simulink model "LabFabSim2022a__10_6_2023"  (R2022a)
settings: Solver=VariableStepAuto  StartTime=0.0  StopTime=400  RelTol=1e-3  EnableMultiTasking=on
model workspace (MAT data in the model file):
  JsonData = timetable
  JsonData.any.CustomProps = struct()
  JsonData.any.VariableCustomProps = struct()
  JsonData.any.versionSavedFrom = 5
  JsonData.any.minCompatibleVersion = 2
  JsonData.any.incompatibilityMsg = ''
  JsonData.any.arrayProps.Description = ''
  JsonData.any.arrayProps.UserData = []
  JsonData.any.arrayProps.TableCustomProperties = struct()
  JsonData.any.data = {[1; 2; 3; 4; 5; 6; 7; 8; 9]}
  JsonData.any.numDims = 2
  JsonData.any.useVarNamesOrig = 0
  JsonData.any.useDimNamesOrig = 0
  JsonData.any.dimNames = {'Time', 'Variables'}
  JsonData.any.dimNamesOrig = {}
  JsonData.any.varNames = {'PartID'}
  JsonData.any.varNamesOrig = {}
  JsonData.any.numRows = 9
  JsonData.any.numVars = 1
  JsonData.any.varDescriptions = {}
  JsonData.any.varUnits = {}
  JsonData.any.rowTimes = datetime
  JsonData.any.rowTimes.data = [1661950057191; 1661949738947; 1661949738947; 1661949738947; 1661949738947; 1661949738947; 1661949738948; 1661949738948; 1661949738948]
  JsonData.any.varContinuity = {}
  M = Simulink.Parameter
  M.DataType = 'auto'
  M.Complexity = 'real'
  M.Dimensions = [0 0]
  ROS_trigger = 0
  SL_ROS_VariableLengthArrays_MaxSizes.CommonInfo.ArrayTruncateAction = 'EmitWarning'
  SL_ROS_VariableLengthArrays_MaxSizes.MsgTypeMap = containers.Map
  SL_ROS_VariableLengthArrays_MaxSizes.MsgTypeMap.serialization.keys = {'std_msgs/UInt32MultiArray', 'std_msgs/UInt64MultiArray', 'std_msgs/UInt8MultiArray'}
  SL_ROS_VariableLengthArrays_MaxSizes.MsgTypeMap.serialization.values{1}.PropertyName = 'Data'
  SL_ROS_VariableLengthArrays_MaxSizes.MsgTypeMap.serialization.values{1}.DataType = 'uint32'
  SL_ROS_VariableLengthArrays_MaxSizes.MsgTypeMap.serialization.values{1}.MaxLength = 31
  SL_ROS_VariableLengthArrays_MaxSizes.MsgTypeMap.serialization.values{2}.PropertyName = 'Data'
  SL_ROS_VariableLengthArrays_MaxSizes.MsgTypeMap.serialization.values{2}.DataType = 'double'
  SL_ROS_VariableLengthArrays_MaxSizes.MsgTypeMap.serialization.values{2}.MaxLength = 31
  SL_ROS_VariableLengthArrays_MaxSizes.MsgTypeMap.serialization.values{3}.PropertyName = 'Data'
  SL_ROS_VariableLengthArrays_MaxSizes.MsgTypeMap.serialization.values{3}.DataType = 'uint8'
  SL_ROS_VariableLengthArrays_MaxSizes.MsgTypeMap.serialization.values{3}.MaxLength = 5
  SL_ROS_VariableLengthArrays_MaxSizes.MsgTypeMap.serialization.uniformity = 0
  SL_ROS_VariableLengthArrays_MaxSizes.MsgTypeMap.serialization.keyType = 'char'
  SL_ROS_VariableLengthArrays_MaxSizes.MsgTypeMap.serialization.valueType = 'any'
undefined symbols (not defined in the file): DOS, DOSinitGen, DTP, DTPGen, DTPInitGen, EmptyLocFound, InitCobot, InitCobotReturn, InitializeSLD, InitLEGO, InitVGRproc2, m, MC, MCGen, MCInitGen, MO, MOGen, MOInitGen, n, NetScan, NetScanInitGen, OrderGen, Spying, SpyingInitGen, WS, WSGen, WSInitGen
libraries: sldelib x1
(part 1 of 4)
settings Model: SimulationMode=external  ExtModeEnableFloating=off  Creator=ise  LastModifiedBy=zdewardener
settings SolverCC: AutoInsertRateTranBlk=on
settings DataIOCC: ExternalInput=[JsonData]  SaveOutput=off
settings OptimizationCC: DefaultParameterBehavior=Inlined  InlineInvariantSignals=on  EnhancedBackFolding=on  PassReuseOutputArgsAs=Individual arguments  StateBitsets=on  DataBitsets=on  ZeroExternalMemoryAtStartup=off  ZeroInternalMemoryAtStartup=off  NoFixptDivByZeroProtection=on  LifeSpan=1  MaxStackSize=64  OptimizeBlockOrder=speed  DifferentSizesBufferReuse=on  EfficientTunableParamExpr=on
settings DebuggingCC: ParameterTunabilityLossMsg=error  UnconnectedInputMsg=warning  UnconnectedOutputMsg=warning  UnconnectedLineMsg=warning
settings HardwareCC: ProdBitPerPointer=32  ProdBitPerSizeT=32  ProdBitPerPtrDiffT=32  ProdLargestAtomicFloat=None  ProdIntDivRoundTo=Floor  ProdWordSize=32  ProdHWDeviceType=Generic->Custom
settings RTWCC: SystemTargetFile=ert.tlc  HardwareBoard=Robot Operating System (ROS)  TLCOptions=-p0 -aRateBasedStepFcn=0  TemplateMakefile=ert_default_tmf  GenerateReport=on  RTWVerbose=off  Toolchain=Catkin  IncludeHyperlinkInReport=on  LaunchReport=on  DLArmComputeVersion=19.05
settings CodeAppCC: ForceParamTrailComments=on  IgnoreCustomStorageClasses=off  OperatorAnnotations=on  SimulinkDataObjDesc=on  SFDataObjDesc=on  CustomSymbolStrGlobalVar=rt$N$M  CustomSymbolStrType=$N$M  CustomSymbolStrFcn=$N$M$F  CustomSymbolStrMacro=$N$M  InsertBlockDesc=on
settings ERTTargetCC: TargetLangStandard=C99 (ISO)  CodeReplacementLibrary=ISO_C  SuppressErrorStatus=on  SupportAbsoluteTime=off  PurelyIntegerCode=on  SupportNonFinite=off  SupportComplex=off  InlinedParameterPlacement=NonHierarchical  RootIOFormat=Structure reference  ERTCustomFileTemplate=example_file_process.tlc

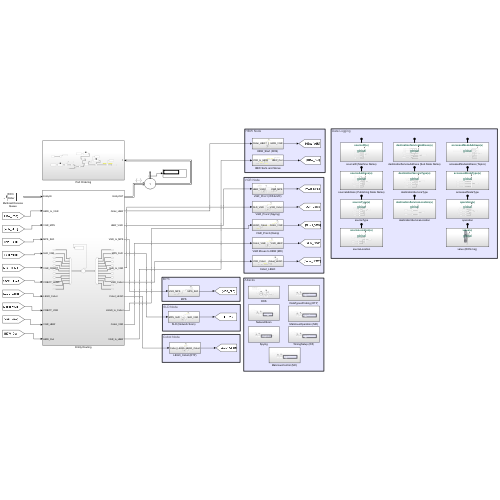
[thumbnail: Simulink's stored preview of the top-level diagram]
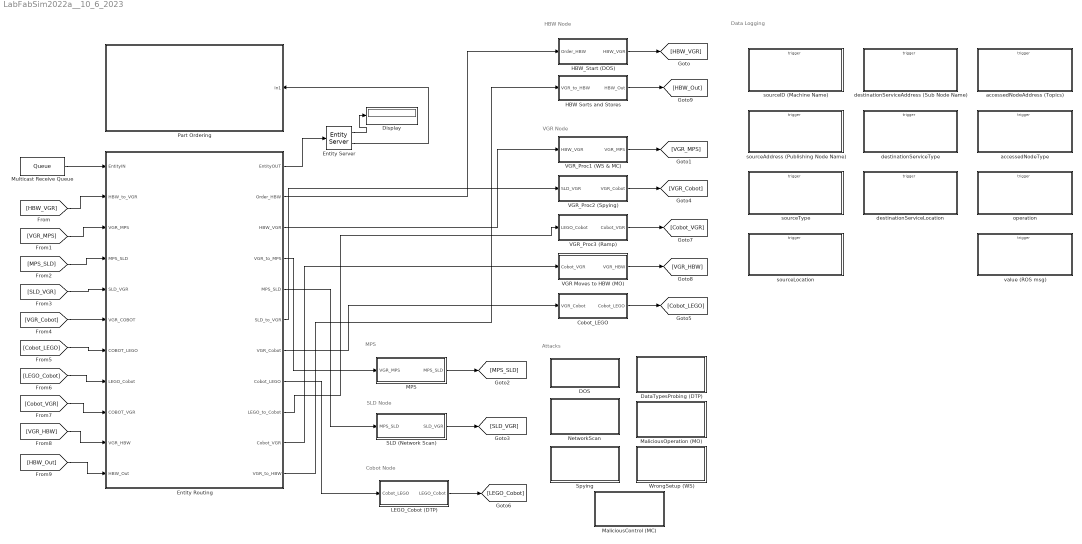
== system LabFabSim2022a__10_6_2023 ==
  note: Attacks
  note: Data Logging
  note: MPS
  note: Cobot Node
  note: SLD Node
  note: VGR Node
  note: HBW Node
  Cobot_LEGO : Subsystem
  DOS : Subsystem
  DataTypesProbing (DTP) : Subsystem
  Display : Display
  Entity Routing : Subsystem
  Entity Server : EntityServer  InputPortMessageModes=m  OutputPortMessageModes=n,m  Capacity=1  EntryAction=|  NumberEntitiesDeparted=on
      | %EntityGen();
      | ReleaseEntity();
      | 
      | entity.CurrentStep = 1;
      | entity.CurrentRoute = 1;
      settings: OutputPortMap=o0,o9
  HBW Sorts and Stores : Subsystem
  HBW_Start (DOS) : Subsystem
  LEGO_Cobot (DTP) : Subsystem
  MPS : Subsystem
  MaliciousControl (MC) : Subsystem
  MaliciousOperation (MO) : Subsystem
  Multicast Receive Queue : Queue  OutputPortMessageModes=m  Capacity=1  EntityArrivalSource=Multicast  MulticastTag=Order
  NetworkScan : Subsystem
  Part Ordering : Subsystem
      settings: PortSchema="{\"entries\":[{\"content\":{\"sides\":[{\"content\":{\"connectorIds\":[]},\"type\":\"ConnectorPlacement.EquallySpacedRectSide\",\"uuid\":\"e994c97d-fb45-4def-b0cb-77e379a9fe28\"},{\"content\":{\"connectorIds\":[\"In1\"],\"side\":\"RIGHT\"},\"type\":\"ConnectorPlacement.EquallySpacedRectSide\",\"uuid\":\"06ce1dc3-22b9-49bf-9481-b353835a56bd\"},{\"content\":{\"connectorIds\":[],\"side\":\"TOP\"},\"type\":\"ConnectorPlacement.EquallySpacedRectSide\",\"uuid\":\"0c5932e5-656f-479c-b83f-b876107c2f45\"}]},\"type\":\"ConnectorPlacement.EquallySpacedConnector\",\"uuid\":\"592d17c9-c3fc-48ea-a782-1c7751a95675\"}],\"packageUris\":[\"http://schema.mathworks.com/mf0/Connector/R2020b\"],\"version\":\"1.0\"}"
  SLD (Network Scan) : Subsystem
  Spying : Subsystem
  VGR Moves to HBW (MO) : Subsystem
  VGR_Proc1 (WS & MC) : Subsystem
  VGR_Proc2 (Spying) : Subsystem
  VGR_Proc3 (Ramp) : Subsystem
  WrongSetup (WS) : Subsystem
  accessedNodeAddress (Topics) : Subsystem  TreatAsAtomicUnit=on
  accessedNodeType : Subsystem  TreatAsAtomicUnit=on
  destinationServiceAddress (Sub Node Name) : Subsystem  TreatAsAtomicUnit=on
  destinationServiceLocation : Subsystem  TreatAsAtomicUnit=on
  destinationServiceType : Subsystem  TreatAsAtomicUnit=on
  operation : Subsystem  TreatAsAtomicUnit=on
  sourceAddress (Publishing Node Name) : Subsystem  TreatAsAtomicUnit=on
  sourceID (Machine Name) : Subsystem  TreatAsAtomicUnit=on
  sourceLocation : Subsystem  TreatAsAtomicUnit=on
  sourceType : Subsystem  TreatAsAtomicUnit=on
  value (ROS msg) : Subsystem  TreatAsAtomicUnit=on
  wires:
  Entity Server/1 -> Display/1
  [HBW_VGR] -> Entity Routing/2(HBW_to_VGR)
  [VGR_MPS] -> Entity Routing/3(VGR_MPS)
  [MPS_SLD] -> Entity Routing/4(MPS_SLD)
  [SLD_VGR] -> Entity Routing/5(SLD_VGR)
  [VGR_Cobot] -> Entity Routing/6(VGR_COBOT)
  [Cobot_LEGO] -> Entity Routing/7(COBOT_LEGO)
  Entity Routing/2(Order_HBW) -> HBW_Start (DOS)/1(Order_HBW)
  Entity Routing/4(VGR_to_MPS) -> MPS/1(VGR_MPS)
  Entity Routing/5("MPS_SLD ") -> SLD (Network Scan)/1(MPS_SLD)
  Entity Routing/6(SLD_to_VGR) -> VGR_Proc2 (Spying)/1(SLD_VGR)
  Entity Routing/7(VGR_Cobot) -> Cobot_LEGO/1(VGR_Cobot)
  HBW_Start (DOS)/1(HBW_VGR) -> [HBW_VGR]
  MPS/1(MPS_SLD) -> [MPS_SLD]
  SLD (Network Scan)/1(SLD_VGR) -> [SLD_VGR]
  VGR_Proc2 (Spying)/1(VGR_Cobot) -> [VGR_Cobot]
  Cobot_LEGO/1(Cobot_LEGO) -> [Cobot_LEGO]
  Entity Routing/3("HBW_VGR ") -> VGR_Proc1 (WS & MC)/1(HBW_VGR)
  VGR_Proc1 (WS & MC)/1(VGR_MPS) -> [VGR_MPS]
  Entity Routing/8(Cobot_LEGO) -> LEGO_Cobot (DTP)/1(Cobot_LEGO)
  [LEGO_Cobot] -> Entity Routing/8(LEGO_Cobot)
  LEGO_Cobot (DTP)/1(LEGO_Cobot) -> [LEGO_Cobot]
  Entity Routing/9(LEGO_to_Cobot) -> VGR_Proc3 (Ramp)/1(LEGO_Cobot)
  VGR_Proc3 (Ramp)/1(Cobot_VGR) -> [Cobot_VGR]
  [Cobot_VGR] -> Entity Routing/9(COBOT_VGR)
  Entity Routing/10(Cobot_VGR) -> VGR Moves to HBW (MO)/1(Cobot_VGR)
  [VGR_HBW] -> Entity Routing/10(VGR_HBW)
  VGR Moves to HBW (MO)/1(VGR_HBW) -> [VGR_HBW]
  Entity Routing/11(VGR_to_HBW) -> HBW Sorts and Stores/1(VGR_to_HBW)
  [HBW_Out] -> Entity Routing/11(HBW_Out)
  HBW Sorts and Stores/1(HBW_Out) -> [HBW_Out]
  Entity Server/2 -> Part Ordering/1(In1)
  Entity Routing/1(EntityOUT) -> Entity Server/1
  Multicast Receive Queue/1 -> Entity Routing/1(EntityIN)

== system LabFabSim2022a__10_6_2023/Cobot_LEGO ==
  note: Calling cobot for picking
  note: Order is ready for pickup
  VGR_Cobot : Inport
  Cobot moving to pickup loc : EntityServer  InputPortMessageModes=m  OutputPortMessageModes=m  Capacity=1  ServiceTimeSource=MATLAB action  ServiceTimeValue=0.1  ServiceTimeAction=|  EntryAction=|  ExitAction=|
      ServiceTimeAction=|
      | dt=0
      | persistent rngInit;
      | if isempty(rngInit)
      |     seed = entity.Rand_seed;
      |     rng(seed);
      |     rngInit = true;
      | end
      | 
      | if entity.ColorID == 1 %red
      |     % Pattern: Uniform distribution
      |     % m: Minimum, M: Maximum
      |     m = 0.2372; M = 0.2624;
      |     dt = m + (M - m) * rand;
      | elseif entity.ColorID == 2 %blue
      |     m = 0.1684; M = 0.2499;
      |     dt = m + (M - m) * rand;
      | elseif entity.ColorID == 3 %white
      |     m = 0.2056; M = 0.2679;
      |     dt = m + (M - m) * rand;
      | end
      EntryAction=|
      | sourceID(6); %cobot
      | sourceAddress(5); %/listener(cobot)
      | sourceType(1); %motion sensor
      | sourceLocation(1); %Fischertechnik
      | destinationServiceAddress(3); %/status_update(main)?
      | destinationServiceType(5); %Next task
      | destinationServiceLocation(2); %Expansion
      | accessedNodeAddress(5); 
      | accessedNodeType(2); %Boolean
      | operation(3); %notify-callback
      | value(34); %Order is ready for pickup
      ExitAction=|
      | sourceID(2); %vgr
      | sourceAddress(2); %/vgr_node
      | sourceType(1); %motion sensor
      | sourceLocation(1); %Fischertechnik
      | destinationServiceAddress(5); %/listener(cobot)
      | destinationServiceType(5); %next task
      | destinationServiceLocation(2); %Expansion
      | accessedNodeAddress(3); 
      | accessedNodeType(1); %String
      | operation(3); %notify-callback
      | value(33); %Calling cobot for picking
  Entity Gate : EntityGate  InputPortMessageModes=m,m  OutputPortMessageModes=m  OperatingMode=Release gate
  Entity Server : EntityServer  InputPortMessageModes=m  OutputPortMessageModes=m  Capacity=1  ServiceTimeSource=MATLAB action  ServiceTimeAction=|
      | dt=0
      | persistent rngInit;
      | if isempty(rngInit)
      |     seed = entity.Rand_seed;
      |     rng(seed);
      |     rngInit = true;
      | end
      | 
      | if entity.ColorID == 1 %red
      |     % Pattern: Uniform distribution
      |     % m: Minimum, M: Maximum
      |     m = 0.0028; M = 0.01;
      |     dt = m + (M - m) * rand;
      | elseif entity.ColorID == 2 %blue
      |     m = 0.007; M = 0.051;
      |     dt = m + (M - m) * rand;
      | elseif entity.ColorID == 3 %white
      |     m = 0.0037; M = 0.0045;
      |     dt = m + (M - m) * rand;
      | end
  Pump off; Return to home pos : EntityServer  InputPortMessageModes=m  OutputPortMessageModes=m  Capacity=1  ServiceTimeValue=5  EntryAction=InitLEGO();
  Pump on; Moving to main LEGO belt : EntityServer  InputPortMessageModes=m  OutputPortMessageModes=m  Capacity=1  ServiceTimeValue=15
  Simulink Function : Subsystem  TreatAsAtomicUnit=on
  Cobot_LEGO : Outport
  wires:
  VGR_Cobot/1 -> Entity Server/1
  Cobot moving to pickup loc/1 -> Pump on; Moving to main LEGO belt/1
  Pump on; Moving to main LEGO belt/1 -> Pump off; Return to home pos/1
  Pump off; Return to home pos/1 -> Entity Gate/2
  Entity Gate/1 -> Cobot_LEGO/1
  Simulink Function/1(Out1) -> Entity Gate/1
  Entity Server/1 -> Cobot moving to pickup loc/1

== system LabFabSim2022a__10_6_2023/DOS ==
  note: Entity Gate:
      | set to open when a positive signal value is passed into the control port. Closes when negative.
  note: Generates a single entity that causes DOSattack (entity generator) to generate 400 entities for DOS attack
  note: Sets DOS_id up to 400 and resets to 1 for next DOS attack
  note: On Service Completion: Send a signal to data-logging SimFunctions
  note: Service Time: 1 Timestep
  note: Recieve signal from Chance-setting Server block for activation signal
  DOS : Subsystem  TreatAsAtomicUnit=on
  Display : Display
  Entity Gate : EntityGate  InputPortMessageModes=m,m  OutputPortMessageModes=m
  Entity Generator : EntityGenerator  InputPortMessageModes=m  OutputPortMessageModes=m  GenerationMethod=Event-based  IntergenerationTimeAction=|  GenerateAction=|  AttributeName=DOS_id  EntityType=Structured  EntityTypeName=DOSattack
      IntergenerationTimeAction=|
      | chanceDOS = rand(1,1);
      | if chanceDOS < 0.3
      |     dt = 1
      GenerateAction=|
      | persistent next_id_DOS
      | 
      | if isempty(next_id_DOS)
      |     next_id_DOS = 1;
      |     %set seed for random number generation
      |     rng(12345);
      | end
      | 
      | entity.DOS_id = next_id_DOS
      | next_id_DOS = next_id_DOS + 1
      | 
      | if entity.DOS_id == 400
      |     next_id_DOS = 1
      settings: InputPortMap=u0
  Entity Server : EntityServer  InputPortMessageModes=m  OutputPortMessageModes=m  Capacity=1  ServiceTimeValue=1  ServiceCompleteAction=|
      | sourceID(3); %main
      | sourceAddress(6); %/order
      | sourceType(4); %order
      | sourceLocation(3); %SCADA system
      | destinationServiceAddress(1); %/hbw_node
      | destinationServiceType(4); %order
      | destinationServiceLocation(1); %Fischertechnik
      | accessedNodeAddress(1); 
      | accessedNodeType(1); %String
      | operation(3); %notify-callback
      | value(1); %hbw recieved an order
  Entity Store : EntityStore  InputPortMessageModes=m  OutputPortMessageModes=m  Capacity=401
      settings: OutputPortMap=o4
  Entity Terminator1 : EntityTerminator  InputPortMessageModes=m  NumberEntitiesArrived=on
      settings: OutputPortMap=o0
  InitDOS : Subsystem
  "Number of Entities Generated from main " : Display
  Simulink Function1 : Subsystem  TreatAsAtomicUnit=on
  Subsystem1 : Subsystem
  wires:
  InitDOS/1(Out1) -> "Number of Entities Generated from main "/1
  Subsystem1/1(Out1) -> Simulink Function1/1(In1)
  DOS/1(Out1) -> Entity Gate/1
  Entity Gate/1 -> Entity Server/1
  Entity Generator/1 -> Entity Store/1
  Entity Server/1 -> Entity Terminator1/1
  Simulink Function1/1(Out1) -> Entity Generator/1
  Entity Store/1 -> Entity Gate/2
  Entity Terminator1/1 -> Display/1

== system LabFabSim2022a__10_6_2023/DataTypesProbing (DTP) ==
  note: SourID(5), SourAdd(4), SourType(1), SourLoc(2), Dest.Serv.Add(5), Dest.Serv.Type(5), Dest.Serv.Loc(2), Acc.Node.Add(4), Acc.Node.Type(1,3), Op(1), Val(46)
  note: Entity Gate:
      | set to open when a positive signal value is passed into the control port. Closes when negative.
  note: Recieve signal from Chance-setting Server block for activation signal
  note: Service Time: 1000 Timestep
  note: Generates a single entity that causes Spying attack (entity generator) to generate one entity
  note: Sets DTP_id up to 6 and resets to 1 for next DataTypesProbing attack
  note: On Service Completion: Send a signal to data-logging SimFunctions
  note: Service Time: 310 Timestep
  Display : Display
  Entity Gate : EntityGate  InputPortMessageModes=m,m  OutputPortMessageModes=m
  Entity Generator : EntityGenerator  InputPortMessageModes=m  OutputPortMessageModes=m  GenerationMethod=Event-based  IntergenerationTimeAction=|  GenerateAction=|  AttributeName=DTP_id  EntityType=Structured  EntityTypeName=DTPAttack
      IntergenerationTimeAction=|
      | chanceDOS = rand(1,1);
      | if chanceDOS < 0.3
      |     dt = 1
      GenerateAction=|
      | persistent next_id_DTP
      | 
      | if isempty(next_id_DTP)
      |     next_id_DTP = 1;
      |     %set seed for random number generation
      |     rng(12345);
      | end
      | 
      | entity.DTP_id = next_id_DTP
      | next_id_DTP = next_id_DTP + 1
      | 
      | if entity.DTP_id == 1
      |     next_id_DTP = 1
      settings: InputPortMap=u0
  Entity Server : EntityServer  InputPortMessageModes=m  OutputPortMessageModes=m  Capacity=1  ServiceTimeValue=1000  ServiceCompleteAction=|
      | sourceID(5); %Lego
      | sourceAddress(1); %/lego_node
      | sourceType(1); %motion Sensor
      | sourceLocation(2); %Expansion
      | destinationServiceAddress(5); %/listener(cobot)
      | destinationServiceType(5); %Next Task
      | destinationServiceLocation(2); %Expansion
      | accessedNodeAddress(4); 
      | accessedNodeType(1); %String
      | operation(1); %read/write
      | value(46); %DTP
  Entity Server1 : EntityServer  InputPortMessageModes=m  OutputPortMessageModes=m  Capacity=1  ServiceTimeValue=310  ServiceCompleteAction=|
      | sourceID(5); %Lego
      | sourceAddress(1); %/lego_node
      | sourceType(1); %motion Sensor
      | sourceLocation(2); %Expansion
      | destinationServiceAddress(5); %/listener(cobot)
      | destinationServiceType(5); %Next Task
      | destinationServiceLocation(2); %Expansion
      | accessedNodeAddress(4); 
      | accessedNodeType(3); %Integer
      | operation(1); %read/write
      | value(46); %DTP
  Entity Store : EntityStore  InputPortMessageModes=m  OutputPortMessageModes=m  Capacity=2
      settings: OutputPortMap=o4
  Entity Terminator1 : EntityTerminator  InputPortMessageModes=m  NumberEntitiesArrived=on
      settings: OutputPortMap=o0
  InitDataTypesProbing : Subsystem
  "Number of Entities Generated from main " : Display
  Simulink Function1 : Subsystem  TreatAsAtomicUnit=on
  Spying : Subsystem  TreatAsAtomicUnit=on
  Subsystem1 : Subsystem
  wires:
  Simulink Function1/1(Out1) -> Entity Generator/1
  Entity Terminator1/1 -> Display/1
  Entity Generator/1 -> Entity Store/1
  Entity Store/1 -> Entity Gate/2
  Entity Server/1 -> Entity Server1/1
  Spying/1(Out1) -> Entity Gate/1
  Subsystem1/1(Out1) -> Simulink Function1/1(In1)
  InitDataTypesProbing/1(Out1) -> "Number of Entities Generated from main "/1
  Entity Server1/1 -> Entity Terminator1/1
  Entity Gate/1 -> Entity Server/1

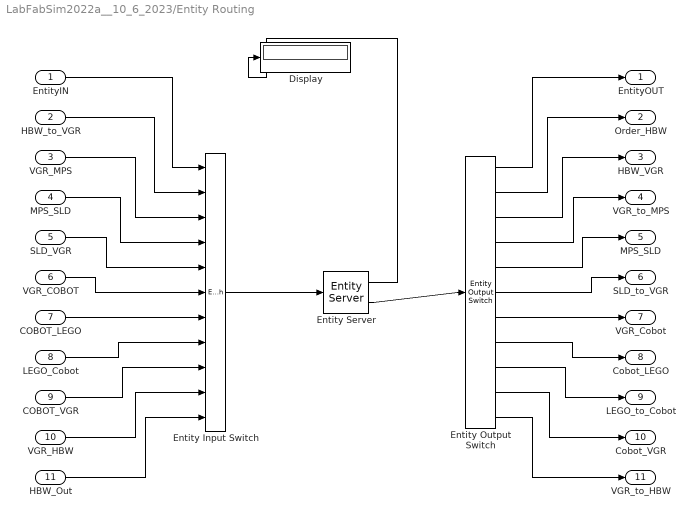
== system LabFabSim2022a__10_6_2023/Entity Routing ==
  EntityIN : Inport
  HBW_to_VGR : Inport  Port=2
  VGR_MPS : Inport  Port=3
  MPS_SLD : Inport  Port=4
  SLD_VGR : Inport  Port=5
  VGR_COBOT : Inport  Port=6
  COBOT_LEGO : Inport  Port=7
  LEGO_Cobot : Inport  Port=8
  COBOT_VGR : Inport  Port=9
  VGR_HBW : Inport  Port=10
  HBW_Out : Inport  Port=11
  Display : Display
  Entity Input Switch : EntityInputSwitch  InputPortMessageModes=m,m,m,m,m,m,m,m,m,m,m  OutputPortMessageModes=m  NumberInputPorts=11
      settings: InputPortMap=u1,u2,u3,u4,u5,u6,u7,u8,u9,u10,u11
  Entity Output Switch : EntityOutputSwitch  InputPortMessageModes=m  OutputPortMessageModes=m,m,m,m,m,m,m,m,m,m,m  NumberOutputPorts=11  SwitchingCriterion=From attribute  SwitchAttributeName=CurrentRoute
      settings: OutputPortMap=o0,o1,o2,o3,o4,o5,o6,o7,o8,o9,o10
  Entity Server : EntityServer  InputPortMessageModes=m  OutputPortMessageModes=n,m  Capacity=1  ServiceTimeValue=0  EntryAction=|  NumberEntitiesDeparted=on
      | entity.CurrentRoute = entity.ServiceProcess(entity.CurrentStep);
      | entity.CurrentStep = entity.CurrentStep + 1;
      settings: OutputPortMap=o0,o9
  EntityOUT : Outport
  Order_HBW : Outport  Port=2
  "HBW_VGR " : Outport  Port=3
  VGR_to_MPS : Outport  Port=4
  "MPS_SLD " : Outport  Port=5
  SLD_to_VGR : Outport  Port=6
  VGR_Cobot : Outport  Port=7
  Cobot_LEGO : Outport  Port=8
  LEGO_to_Cobot : Outport  Port=9
  Cobot_VGR : Outport  Port=10
  VGR_to_HBW : Outport  Port=11
  wires:
  EntityIN/1 -> Entity Input Switch/1
  HBW_to_VGR/1 -> Entity Input Switch/2
  VGR_MPS/1 -> Entity Input Switch/3
  MPS_SLD/1 -> Entity Input Switch/4
  SLD_VGR/1 -> Entity Input Switch/5
  VGR_COBOT/1 -> Entity Input Switch/6
  COBOT_LEGO/1 -> Entity Input Switch/7
  Entity Input Switch/1 -> Entity Server/1
  Entity Server/2 -> Entity Output Switch/1
  Entity Output Switch/1 -> EntityOUT/1
  Entity Output Switch/2 -> Order_HBW/1
  Entity Output Switch/3 -> "HBW_VGR "/1
  Entity Output Switch/4 -> VGR_to_MPS/1
  Entity Output Switch/5 -> "MPS_SLD "/1
  Entity Output Switch/6 -> SLD_to_VGR/1
  Entity Output Switch/7 -> VGR_Cobot/1
  Entity Server/1 -> Display/1
  Entity Output Switch/8 -> Cobot_LEGO/1
  Entity Output Switch/9 -> LEGO_to_Cobot/1
  Entity Output Switch/10 -> Cobot_VGR/1
  Entity Output Switch/11 -> VGR_to_HBW/1
  LEGO_Cobot/1 -> Entity Input Switch/8
  COBOT_VGR/1 -> Entity Input Switch/9
  VGR_HBW/1 -> Entity Input Switch/10
  HBW_Out/1 -> Entity Input Switch/11

== system LabFabSim2022a__10_6_2023/HBW Sorts and Stores ==
  note: HBW Robot is Set to Home
  note: Status updated successfully
  note: HBW Placed Material on the Shelf
  note: VGR is Set to Home
  note: HBW Picked up Material from the Belt
  note: Material is Ready for HBW Pick Up
  VGR_to_HBW : Inport
  Entity Server : EntityServer  InputPortMessageModes=m  OutputPortMessageModes=m  Capacity=1  ServiceTimeSource=MATLAB action  ServiceTimeAction=|
      | dt=0
      | persistent rngInit;
      | if isempty(rngInit)
      |     seed = entity.Rand_seed;
      |     rng(seed);
      |     rngInit = true;
      | end
      | 
      | if entity.ColorID == 1 %red
      |     % Pattern: Uniform distribution
      |     % m: Minimum, M: Maximum
      |     m = 1.9949; M = 1.9965;
      |     dt = m + (M - m) * rand;
      | elseif entity.ColorID == 2 %blue
      |     m = 1.9508; M = 1.9938;
      |     dt = m + (M - m) * rand;
      | elseif entity.ColorID == 3 %white
      |     m = 1.8972; M = 1.9967;
      |     dt = m + (M - m) * rand;
      | end
  Entity Server1 : EntityServer  InputPortMessageModes=m  OutputPortMessageModes=m  Capacity=1  ServiceTimeSource=MATLAB action  ServiceTimeAction=|
      | dt=0
      | persistent rngInit;
      | if isempty(rngInit)
      |     seed = entity.Rand_seed;
      |     rng(seed);
      |     rngInit = true;
      | end
      | 
      | if entity.ColorID == 1 %red
      |     % Pattern: Uniform distribution
      |     % m: Minimum, M: Maximum
      |     m = 19.7937; M = 19.8988;
      |     dt = m + (M - m) * rand;
      | elseif entity.ColorID == 2 %blue
      |     m = 16.4596; M = 16.7641;
      |     dt = m + (M - m) * rand;
      | elseif entity.ColorID == 3 %white
      |     m = 23.1035; M = 23.7903;
      |     dt = m + (M - m) * rand;
      | end
  HBW Sorting and updating json file : EntityServer  InputPortMessageModes=m  OutputPortMessageModes=m  Capacity=1  ServiceTimeSource=MATLAB action  ServiceTimeValue=0.5  ServiceTimeAttributeName=HBW_ServiceTime  ServiceTimeAction=|  EntryAction=|  ExitAction=|
      ServiceTimeAction=|
      | dt=0
      | persistent rngInit;
      | if isempty(rngInit)
      |     seed = entity.Rand_seed;
      |     rng(seed);
      |     rngInit = true;
      | end
      | 
      | if entity.ColorID == 1 %red
      |     % Pattern: Uniform distribution
      |     % m: Minimum, M: Maximum
      |     m = 0.0103; M = 0.0276;
      |     dt = m + (M - m) * rand;
      | elseif entity.ColorID == 2 %blue
      |     m = 0.0071; M = 0.0138;
      |     dt = m + (M - m) * rand;
      | elseif entity.ColorID == 3 %white
      |     m = 0.014; M = 0.0204;
      |     dt = m + (M - m) * rand;
      | end
      EntryAction=|
      | sourceID(1); %hbw
      | sourceAddress(1); %/hbw_node
      | sourceType(5); %next task
      | sourceLocation(1); %Fischertechnik
      | destinationServiceAddress(3); %/status_update
      | destinationServiceType(5); %next task
      | destinationServiceLocation(1); %Fischertechnik
      | accessedNodeAddress(1); 
      | accessedNodeType(1); %String
      | operation(3); %notify-callback
      | value(14); %hbw empty box is back on the shelf
      ExitAction=|
      | sourceID(1); %hbw
      | sourceAddress(1); %/hbw_node
      | sourceType(5); %next task
      | sourceLocation(1); %Fischertechnik
      | destinationServiceAddress(3); %/status_update
      | destinationServiceType(5); %next task
      | destinationServiceLocation(1); %Fischertechnik
      | accessedNodeAddress(6); 
      | accessedNodeType(1); %String
      | operation(3); %notify-callback
      | value(42); %Status Updated Successfully
  HBW returns home : EntityServer  InputPortMessageModes=m  OutputPortMessageModes=m  Capacity=1  ServiceTimeSource=MATLAB action  ServiceTimeValue=20  ServiceTimeAttributeName=HBW_ServiceTime  ServiceTimeAction=|  ExitAction=|
      ServiceTimeAction=|
      | dt=0
      | persistent rngInit;
      | if isempty(rngInit)
      |     seed = entity.Rand_seed;
      |     rng(seed);
      |     rngInit = true;
      | end
      | 
      | if entity.ColorID == 1 %red
      |     % Pattern: Uniform distribution
      |     % m: Minimum, M: Maximum
      |     m = 14.049; M = 14.2335;
      |     dt = m + (M - m) * rand;
      | elseif entity.ColorID == 2 %blue
      |     m = 10.9437; M = 11.1714;
      |     dt = m + (M - m) * rand;
      | elseif entity.ColorID == 3 %white
      |     m = 17.375; M = 17.9006;
      |     dt = m + (M - m) * rand;
      | end
      ExitAction=|
      | sourceID(1); %hbw
      | sourceAddress(1); %/hbw_node
      | sourceType(3); %reference switch
      | sourceLocation(1); %Fischertechnik
      | destinationServiceAddress(3); %/status_update
      | destinationServiceType(5); %next task
      | destinationServiceLocation(1); %Fischertechnik
      | accessedNodeAddress(1); 
      | accessedNodeType(1); %String
      | operation(3); %notify-callback
      | value(15); %hbw robot is set to home
  "HBW-side light gate " : EntityServer  InputPortMessageModes=m  OutputPortMessageModes=m  Capacity=1  ServiceTimeSource=MATLAB action  ServiceTimeValue=0.5  ServiceTimeAttributeName=HBW_ServiceTime  ServiceTimeAction=|  EntryAction=|  ExitAction=|
      ServiceTimeAction=|
      | dt=0
      | persistent rngInit;
      | if isempty(rngInit)
      |     seed = entity.Rand_seed;
      |     rng(seed);
      |     rngInit = true;
      | end
      | 
      | if entity.ColorID == 1 %red
      |     % Pattern: Uniform distribution
      |     % m: Minimum, M: Maximum
      |     m = 0.5351; M = 0.5768;
      |     dt = m + (M - m) * rand;
      | elseif entity.ColorID == 2 %blue
      |     m = 0.5457; M = 0.5946;
      |     dt = m + (M - m) * rand;
      | elseif entity.ColorID == 3 %white
      |     m = 0.5429; M = 0.5509;
      |     dt = m + (M - m) * rand;
      | end
      EntryAction=|
      | sourceID(1); %hbw
      | sourceAddress(1); %/hbw_node
      | sourceType(1); %Motion Sensor
      | sourceLocation(1); %Fischertechnik
      | destinationServiceAddress(1); %/hbw_node
      | destinationServiceType(5); %next task
      | destinationServiceLocation(1); %Fischertechnik
      | accessedNodeAddress(1); 
      | accessedNodeType(2); %Boolean
      | operation(3); %notify-callback
      | value(10); %Material is Ready for HBW Pick Up
      ExitAction=|
      | sourceID(1); %hbw
      | sourceAddress(1); %/hbw_node
      | sourceType(1); %Motion Sensor
      | sourceLocation(1); %Fischertechnik
      | destinationServiceAddress(1); %/hbw_node
      | destinationServiceType(5); %next task
      | destinationServiceLocation(1); %Fischertechnik
      | accessedNodeAddress(1); 
      | accessedNodeType(2); %Boolean
      | operation(3); %notify-callback
      | value(12); %HBW Picked up Material from the Belt
  VGR returns home : EntityServer  InputPortMessageModes=m  OutputPortMessageModes=m  Capacity=1  ServiceTimeSource=MATLAB action  ServiceTimeValue=1.7  ServiceTimeAttributeName=HBW_ServiceTime  ServiceTimeAction=|  ServiceCompleteAction=|
      ServiceTimeAction=|
      | dt=0
      | persistent rngInit;
      | if isempty(rngInit)
      |     seed = entity.Rand_seed;
      |     rng(seed);
      |     rngInit = true;
      | end
      | 
      | if entity.ColorID == 1 %red
      |     % Pattern: Uniform distribution
      |     % m: Minimum, M: Maximum
      |     m = 1.4321; M = 1.478;
      |     dt = m + (M - m) * rand;
      | elseif entity.ColorID == 2 %blue
      |     m = 1.3652; M = 1.4388;
      |     dt = m + (M - m) * rand;
      | elseif entity.ColorID == 3 %white
      |     m = 1.3846; M = 1.45;
      |     dt = m + (M - m) * rand;
      | end
      ServiceCompleteAction=|
      | sourceID(2); %vgr
      | sourceAddress(2); %/vgr_node
      | sourceType(5); %next task
      | sourceLocation(1); %Fischertechnik
      | destinationServiceAddress(2); %/vgr_node
      | destinationServiceType(3); %reference switch
      | destinationServiceLocation(1); %Fischertechnik
      | accessedNodeAddress(3); 
      | accessedNodeType(1); %String
      | operation(3); %notify-callback
      | value(16); %vgr is set to home
  HBW_Out : Outport
  wires:
  VGR_to_HBW/1 -> Entity Server/1
  "HBW-side light gate "/1 -> VGR returns home/1
  Entity Server/1 -> "HBW-side light gate "/1
  VGR returns home/1 -> Entity Server1/1
  HBW Sorting and updating json file/1 -> HBW returns home/1
  HBW returns home/1 -> HBW_Out/1
  Entity Server1/1 -> HBW Sorting and updating json file/1

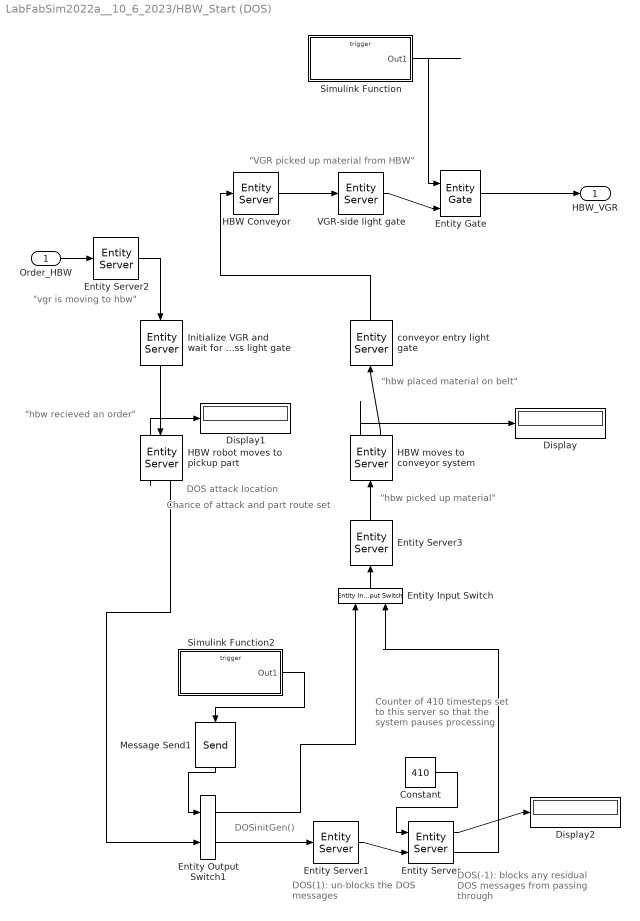
== system LabFabSim2022a__10_6_2023/HBW_Start (DOS) ==
  note: Chance of attack and part route set
  note: Counter of 410 timesteps set to this server so that the system pauses processing
  note: DOS(-1):
      | blocks any residual DOS messages from passing through
  note: DOS(1):
      | un-blocks the DOS messages
  note: "vgr is moving to hbw"
  note: "VGR picked up material from HBW"
  note: "hbw placed material on belt"
  note: "hbw picked up material"
  note: "hbw recieved an order"
  note: DOS attack location
  note: DOSinitGen()
  Order_HBW : Inport
  Constant : Constant  Value=410
  Display : Display
  Display1 : Display
  Display2 : Display
  Entity Input Switch : EntityInputSwitch  InputPortMessageModes=m,m  OutputPortMessageModes=m
  Entity Output Switch1 : EntityOutputSwitch  InputPortMessageModes=m,m  OutputPortMessageModes=m,m  SwitchingCriterion=From control port  SwitchAttributeName=Attribute1
      settings: InputPortMap=u0,u1
  Entity Gate : EntityGate  InputPortMessageModes=m,m  OutputPortMessageModes=m  OperatingMode=Release gate
  Entity Server : EntityServer  InputPortMessageModes=n,m  OutputPortMessageModes=n,m  Capacity=1  ServiceTimeSource=Signal port  ExitAction=DOS(-1);  NumberEntitiesDeparted=on
      settings: InputPortMap=u0,u2  OutputPortMap=o0,o9
  Entity Server1 : EntityServer  InputPortMessageModes=m  OutputPortMessageModes=m  Capacity=1  EntryAction=DOSinitGen();  ServiceCompleteAction=DOS(1);
  Entity Server2 : EntityServer  InputPortMessageModes=m  OutputPortMessageModes=m  Capacity=1  ServiceTimeSource=MATLAB action  ServiceTimeAction=|
      | dt=0
      | persistent rngInit;
      | if isempty(rngInit)
      |     seed = entity.Rand_seed;
      |     rng(seed);
      |     rngInit = true;
      | end
      | 
      | if entity.ColorID == 1 %red
      |     % Pattern: Uniform distribution
      |     % m: Minimum, M: Maximum
      |     m = 0.01819; M = 0.11747;
      |     dt = m + (M - m) * rand;
      | elseif entity.ColorID == 2 %blue
      |     m = 0.00819; M = 0.10134;
      |     dt = m + (M - m) * rand;
      | elseif entity.ColorID == 3 %white
      |     m = 0.00559; M = 0.05693;
      |     dt = m + (M - m) * rand;
      | end
  Entity Server3 : EntityServer  InputPortMessageModes=m  OutputPortMessageModes=m  Capacity=1  ServiceTimeSource=MATLAB action  ServiceTimeAction=|
      | dt=0
      | persistent rngInit;
      | if isempty(rngInit)
      |     seed = entity.Rand_seed;
      |     rng(seed);
      |     rngInit = true;
      | end
      | 
      | if entity.ColorID == 1 %red
      |     % Pattern: Uniform distribution
      |     % m: Minimum, M: Maximum
      |     m = 13.81674; M = 15.52105;
      |     dt = m + (M - m) * rand;
      | elseif entity.ColorID == 2 %blue
      |     m = 10.68302; M = 10.81544;
      |     dt = m + (M - m) * rand;
      | elseif entity.ColorID == 3 %white
      |     m = 17.46035; M = 18.19719;
      |     dt = m + (M - m) * rand;
      | end
  HBW Conveyor : EntityServer  InputPortMessageModes=m  OutputPortMessageModes=m  Capacity=1  ServiceTimeSource=MATLAB action  ServiceTimeAction=|
      | dt=0
      | persistent rngInit;
      | if isempty(rngInit)
      |     seed = entity.Rand_seed;
      |     rng(seed);
      |     rngInit = true;
      | end
      | 
      | if entity.ColorID == 1 %red
      |     % Pattern: Uniform distribution
      |     % m: Minimum, M: Maximum
      |     m = 4.91336; M = 4.93075;
      |     dt = m + (M - m) * rand;
      | elseif entity.ColorID == 2 %blue
      |     m = 5.01319; M = 5.07688;
      |     dt = m + (M - m) * rand;
      | elseif entity.ColorID == 3 %white
      |     m = 4.93141; M = 4.97213;
      |     dt = m + (M - m) * rand;
      | end
  HBW moves to conveyor system : EntityServer  InputPortMessageModes=m  OutputPortMessageModes=n,m  Capacity=1  ServiceTimeSource=MATLAB action  ServiceTimeValue=5  ServiceTimeAttributeName=HBW_ServiceTime  ServiceTimeAction=|  EntryAction=|  NumberEntitiesDeparted=on
      ServiceTimeAction=|
      | dt=0
      | persistent rngInit;
      | if isempty(rngInit)
      |     seed = entity.Rand_seed;
      |     rng(seed);
      |     rngInit = true;
      | end
      | 
      | if entity.ColorID == 1 %red
      |     % Pattern: Uniform distribution
      |     % m: Minimum, M: Maximum
      |     m = 18.6675; M = 20.17508;
      |     dt = m + (M - m) * rand;
      | elseif entity.ColorID == 2 %blue
      |     m = 17.17357; M = 17.69853;
      |     dt = m + (M - m) * rand;
      | elseif entity.ColorID == 3 %white
      |     m = 23.25977; M = 23.95334;
      |     dt = m + (M - m) * rand;
      | end
      EntryAction=|
      | sourceID(1); %hbw
      | sourceAddress(1); %/hbw_node
      | sourceType(3); %reference switch
      | sourceLocation(1); %Fischertechnik
      | destinationServiceAddress(1); %/hbw_node
      | destinationServiceType(5); %next task
      | destinationServiceLocation(1); %Fischertechnik
      | accessedNodeAddress(1); 
      | accessedNodeType(1); %String
      | operation(3); %notify-callback
      | value(3); %hbw picked up materials
      settings: OutputPortMap=o0,o9
  HBW robot moves to pickup part : EntityServer  InputPortMessageModes=m  OutputPortMessageModes=n,m  Capacity=1  ServiceTimeValue=0  ServiceTimeAttributeName=entity  EntryAction=|  ExitAction=|  NumberEntitiesDeparted=on
      EntryAction=|
      | sourceID(3); %main
      | sourceAddress(1); %/hbw_node
      | sourceType(4); %order
      | sourceLocation(3); %SCADA system
      | destinationServiceAddress(1); %/hbw_node
      | destinationServiceType(4); %order
      | destinationServiceLocation(1); %Fischertechnik
      | accessedNodeAddress(1); 
      | accessedNodeType(1); %String
      | operation(3); %notify-callback
      | value(1); %hbw recieved an order
      ExitAction=|
      | chanceDOS = rand(1,1)
      | if chanceDOS < 0.0
      |     %DOS Attack Happening!
      |     DOS_Router(1);
      | 
      | else
      |     %Normal Behavior
      |     DOS(-1);
      |     DOS_Router(2);
      | end
      settings: OutputPortMap=o0,o9
  Initialize VGR and wait for part to cross light gate : EntityServer  InputPortMessageModes=m  OutputPortMessageModes=m  Capacity=1  ServiceTimeSource=MATLAB action  ServiceTimeValue=0.2  ServiceTimeAction=|  EntryAction=|
      ServiceTimeAction=|
      | dt=0
      | persistent rngInit;
      | if isempty(rngInit)
      |     seed = entity.Rand_seed;
      |     rng(seed);
      |     rngInit = true;
      | end
      | 
      | if entity.ColorID == 1 %red
      |     % Pattern: Uniform distribution
      |     % m: Minimum, M: Maximum
      |     m = 0.00869; M = 0.01195;
      |     dt = m + (M - m) * rand;
      | elseif entity.ColorID == 2 %blue
      |     m = 0.00814; M = 0.11476;
      |     dt = m + (M - m) * rand;
      | elseif entity.ColorID == 3 %white
      |     m = 0.00951; M = 0.01176;
      |     dt = m + (M - m) * rand;
      | end
      EntryAction=|
      | sourceID(3); %main
      | sourceAddress(2); %/vgr_node
      | sourceType(5); %next task
      | sourceLocation(1); %Fischer
      | destinationServiceAddress(2); %/vgr_node
      | destinationServiceType(5); %next task
      | destinationServiceLocation(1); %Fischertechnik
      | accessedNodeAddress(3); 
      | accessedNodeType(1); %String
      | operation(3); %notify-callback
      | value(29); %vgr is moving to hbw
  Message Send1 : Send  OutputPortMessageModes=m
  Simulink Function : Subsystem  TreatAsAtomicUnit=on
  Simulink Function2 : Subsystem  TreatAsAtomicUnit=on
  VGR-side light gate : EntityServer  InputPortMessageModes=m  OutputPortMessageModes=m  Capacity=1  ServiceTimeValue=0.1  EntryAction=|
      | VGR_PickupPart();
      | 
      | sourceID(1); %hbw
      | sourceAddress(1); %/hbw_node
      | sourceType(1); %Motion Sensor 
      | sourceLocation(1); %Fischertechnik
      | destinationServiceAddress(2); %/vgr_node
      | destinationServiceType(5); %next task
      | destinationServiceLocation(1); %Fischertechnik
      | accessedNodeAddress(3); 
      | accessedNodeType(2); %Boolean
      | operation(3); %notify-callback
      | value(30); %VGR picked up material from HBW
  conveyor entry light gate : EntityServer  InputPortMessageModes=m  OutputPortMessageModes=m  Capacity=1  ServiceTimeValue=3  EntryAction=|
      | VGR_PickupPart();
      | 
      | sourceID(1); %hbw
      | sourceAddress(1); %/hbw_node
      | sourceType(1); %Motion Sensor
      | sourceLocation(1); %Fischertechnik
      | destinationServiceAddress(1); %/hbw_node
      | destinationServiceType(5); %next task
      | destinationServiceLocation(1); %Fischertechnik
      | accessedNodeAddress(1); 
      | accessedNodeType(1); %String
      | operation(3); %notify-callback
      | value(5); %hbw placed material on belt
  HBW_VGR : Outport
  wires:
  Simulink Function/1(Out1) -> Entity Gate/1
  Entity Gate/1 -> HBW_VGR/1
  HBW moves to conveyor system/2 -> conveyor entry light gate/1
  conveyor entry light gate/1 -> HBW Conveyor/1
  HBW Conveyor/1 -> VGR-side light gate/1
  VGR-side light gate/1 -> Entity Gate/2
  Order_HBW/1 -> Entity Server2/1
  Initialize VGR and wait for part to cross light gate/1 -> HBW robot moves to pickup part/1
  Entity Output Switch1/1 -> Entity Input Switch/1
  HBW moves to conveyor system/1 -> Display/1
  HBW robot moves to pickup part/1 -> Display1/1
  HBW robot moves to pickup part/2 -> Entity Output Switch1/2
  Entity Output Switch1/2 -> Entity Server1/1
  Entity Server/2 -> Entity Input Switch/2
  Entity Input Switch/1 -> Entity Server3/1
  Constant/1 -> Entity Server/1
  Simulink Function2/1(Out1) -> Message Send1/1
  Message Send1/1 -> Entity Output Switch1/1
  Entity Server/1 -> Display2/1
  Entity Server1/1 -> Entity Server/2
  Entity Server2/1 -> Initialize VGR and wait for part to cross light gate/1
  Entity Server3/1 -> HBW moves to conveyor system/1

== system LabFabSim2022a__10_6_2023/LEGO_Cobot (DTP) ==
  note: <color> order is ready for pickup
  note: DTP (1):
      | un-blocks the DataTypesProbing messages
  note: DTP(-1):
      | blocks any residual DataTypesProbing messages from passing through
  note: Counter of 11,311 timesteps set to this server so that the system pauses processing (1/10 of the time taken in DS2OS dataset)
  note: DTP InitGen()
  note: DataTypesProbing attack location
  note: Chance of attack and part route set
  Cobot_LEGO : Inport
  Constant : Constant  Value=1311
  Display2 : Display
  Entity Input Switch : EntityInputSwitch  InputPortMessageModes=m,m  OutputPortMessageModes=m
  Entity Output Switch1 : EntityOutputSwitch  InputPortMessageModes=m,m  OutputPortMessageModes=m,m  SwitchingCriterion=From control port  SwitchAttributeName=Attribute1
      settings: InputPortMap=u0,u1
  Entity Gate : EntityGate  InputPortMessageModes=m,m  OutputPortMessageModes=m  OperatingMode=Release gate
  Entity Server : EntityServer  InputPortMessageModes=m  OutputPortMessageModes=m  Capacity=1  ServiceTimeSource=MATLAB action  ServiceTimeAction=|  EntryAction=InitCobotReturn();  ExitAction=|
      ServiceTimeAction=|
      | dt=0
      | persistent rngInit;
      | if isempty(rngInit)
      |     seed = entity.Rand_seed;
      |     rng(seed);
      |     rngInit = true;
      | end
      | 
      | if entity.ColorID == 1 %red
      |     % Pattern: Uniform distribution
      |     % m: Minimum, M: Maximum
      |     m = 21.275; M = 35.7505;
      |     dt = m + (M - m) * rand;
      | elseif entity.ColorID == 2 %blue
      |     m = 18.0858; M = 20.012;
      |     dt = m + (M - m) * rand;
      | elseif entity.ColorID == 3 %white
      |     m = 20.5412; M = 21.691;
      |     dt = m + (M - m) * rand;
      | end
      ExitAction=|
      | sourceID(5); %lego
      | sourceAddress(4); %/lego_node
      | sourceType(1); %motion sensor
      | sourceLocation(2); %Expansion
      | destinationServiceAddress(5); %/listener(cobot)
      | destinationServiceType(5); %Next task
      | destinationServiceLocation(2); %Expansion
      | accessedNodeAddress(5); 
      | accessedNodeType(2); %Boolean
      | operation(3); %notify-callback
      | 
      | if entity.ColorID == 1
      |     value(35); %RED order is ready for pickup
      | else if entity.ColorID == 2
      |     value(36); %BLUE order is ready for pickup
      | else
      |     value(37);%WHITE order is ready for pickup
      | end
  Entity Server1 : EntityServer  InputPortMessageModes=n,m  OutputPortMessageModes=n,m  Capacity=1  ServiceTimeSource=Signal port  ExitAction=DTP(-1);  NumberEntitiesDeparted=on
      settings: InputPortMap=u0,u2  OutputPortMap=o0,o9
  Entity Server2 : EntityServer  InputPortMessageModes=m  OutputPortMessageModes=m  Capacity=1  EntryAction=DTPInitGen();  ServiceCompleteAction=DTP(1);
  "LEGO sorting process " : EntityServer  InputPortMessageModes=m  OutputPortMessageModes=m  Capacity=1  ServiceTimeSource=Attribute  ServiceTimeAttributeName=LEGO_ServiceTime  ExitAction=|
      | chanceDTP = rand(1,1)
      | if chanceDTP < 0.0
      |     %Attack Happening!
      |     DTP_Router(1);
      | 
      | else
      |     %Normal Behavior
      |     DTP(-1);
      |     DTP_Router(2);
      | end
  Message Send1 : Send  OutputPortMessageModes=m
  Simulink Function : Subsystem  TreatAsAtomicUnit=on
  Simulink Function2 : Subsystem  TreatAsAtomicUnit=on
  LEGO_Cobot : Outport
  wires:
  Cobot_LEGO/1 -> "LEGO sorting process "/1
  Entity Server/1 -> Entity Gate/2
  Entity Gate/1 -> LEGO_Cobot/1
  Simulink Function/1(Out1) -> Entity Gate/1
  Entity Server1/1 -> Display2/1
  Entity Output Switch1/2 -> Entity Server2/1
  Entity Output Switch1/1 -> Entity Input Switch/1
  Message Send1/1 -> Entity Output Switch1/1
  Entity Server1/2 -> Entity Input Switch/2
  Entity Server2/1 -> Entity Server1/2
  Constant/1 -> Entity Server1/1
  Entity Input Switch/1 -> Entity Server/1
  Simulink Function2/1(Out1) -> Message Send1/1
  "LEGO sorting process "/1 -> Entity Output Switch1/2

== system LabFabSim2022a__10_6_2023/MPS ==
  VGR_MPS : Inport
  CNC Processing : EntityServer  InputPortMessageModes=m  OutputPortMessageModes=m  Capacity=1  ServiceTimeValue=4
  Entity Gate : EntityGate  InputPortMessageModes=m,m  OutputPortMessageModes=m  OperatingMode=Release gate
  MPS brings in part for kiln : EntityServer  InputPortMessageModes=m  OutputPortMessageModes=m  Capacity=1  ServiceTimeValue=4
  MiniVGR picks up part and moves to CNC : EntityServer  InputPortMessageModes=m  OutputPortMessageModes=m  Capacity=1  ServiceTimeValue=4
  Part is ejected onto SLD : EntityServer  InputPortMessageModes=m  OutputPortMessageModes=m  Capacity=1  EntryAction=InitializeSLD();
  Simulink Function : Subsystem  TreatAsAtomicUnit=on
  MPS_SLD : Outport
  wires:
  VGR_MPS/1 -> MPS brings in part for kiln/1
  MPS brings in part for kiln/1 -> MiniVGR picks up part and moves to CNC/1
  MiniVGR picks up part and moves to CNC/1 -> CNC Processing/1
  CNC Processing/1 -> Part is ejected onto SLD/1
  Part is ejected onto SLD/1 -> Entity Gate/2
  Entity Gate/1 -> MPS_SLD/1
  Simulink Function/1(Out1) -> Entity Gate/1

== system LabFabSim2022a__10_6_2023/MaliciousControl (MC) ==
  note: SourID(2), SourAdd(2), SourType(5), SourLoc(1), Dest.Serv.Add(5), Dest.Serv.Type(5), Dest.Serv.Loc(2), Acc.Node.Add(4), Acc.Node.Type(1), Op(3), Val(49)
  note: Entity Gate:
      | set to open when a positive signal value is passed into the control port. Closes when negative.
  note: Recieve signal from Chance-setting Server block for activation signal
  note: Service Time: 3000 Timestep
  note: Generates a single entity that causes Malicious Control attack (entity generator) to generate one entity
  note: Sets MC_id up to 1 and resets to 1 for next Malicious Control attack
  note: On Service Completion: Send a signal to data-logging SimFunctions
  note: Service Time: 65 Timestep
  Display : Display
  Entity Gate : EntityGate  InputPortMessageModes=m,m  OutputPortMessageModes=m
  Entity Generator : EntityGenerator  InputPortMessageModes=m  OutputPortMessageModes=m  GenerationMethod=Event-based  IntergenerationTimeAction=|  GenerateAction=|  AttributeName=MC_id  EntityType=Structured  EntityTypeName=MCAttack
      IntergenerationTimeAction=|
      | chanceDOS = rand(1,1);
      | if chanceDOS < 0.3
      |     dt = 1
      GenerateAction=|
      | persistent next_id_MC
      | 
      | if isempty(next_id_MC)
      |     next_id_MC = 1;
      |     %set seed for random number generation
      |     rng(12345);
      | end
      | 
      | entity.MC_id = next_id_MC
      | next_id_MC = next_id_MC + 1
      | 
      | if entity.MC_id == 1
      |     next_id_MC = 1
      settings: InputPortMap=u0
  Entity Server : EntityServer  InputPortMessageModes=m  OutputPortMessageModes=m  Capacity=1  ServiceTimeValue=3000  ServiceCompleteAction=|
      | sourceID(2); %vgr
      | sourceAddress(2); %/vgr_node
      | sourceType(5); %next task
      | sourceLocation(1); %Fischertechnik
      | destinationServiceAddress(5); %/listener (cobot)
      | destinationServiceType(5); %next task
      | destinationServiceLocation(2); %Expansion
      | accessedNodeAddress(4); 
      | accessedNodeType(1); %String
      | operation(3); %notify-callback
      | value(49); %MC
  Entity Server1 : EntityServer  InputPortMessageModes=m  OutputPortMessageModes=m  Capacity=1  ServiceTimeValue=65  ServiceCompleteAction=|
      | sourceID(2); %vgr
      | sourceAddress(2); %/vgr_node
      | sourceType(5); %next task
      | sourceLocation(1); %Fischertechnik
      | destinationServiceAddress(5); %/listener (cobot)
      | destinationServiceType(5); %next task
      | destinationServiceLocation(2); %Expansion
      | accessedNodeAddress(4); 
      | accessedNodeType(1); %String
      | operation(3); %notify-callback
      | value(49); %MC
  Entity Store : EntityStore  InputPortMessageModes=m  OutputPortMessageModes=m  Capacity=2
      settings: OutputPortMap=o4
  Entity Terminator1 : EntityTerminator  InputPortMessageModes=m  NumberEntitiesArrived=on
      settings: OutputPortMap=o0
  InitMaliciousControl : Subsystem
  Malicious Control : Subsystem  TreatAsAtomicUnit=on
  "Number of Entities Generated from main " : Display
  Simulink Function1 : Subsystem  TreatAsAtomicUnit=on
  Subsystem1 : Subsystem
  wires:
  Simulink Function1/1(Out1) -> Entity Generator/1
  Entity Terminator1/1 -> Display/1
  Entity Generator/1 -> Entity Store/1
  Entity Store/1 -> Entity Gate/2
  Entity Server/1 -> Entity Server1/1
  Malicious Control/1(Out1) -> Entity Gate/1
  Subsystem1/1(Out1) -> Simulink Function1/1(In1)
  InitMaliciousControl/1(Out1) -> "Number of Entities Generated from main "/1
  Entity Server1/1 -> Entity Terminator1/1
  Entity Gate/1 -> Entity Server/1

== system LabFabSim2022a__10_6_2023/MaliciousOperation (MO) ==
  note: SourID(2), SourAdd(2), SourType(5), SourLoc(1), Dest.Serv.Add(1), Dest.Serv.Type(1), Dest.Serv.Loc(1), Acc.Node.Add(3), Acc.Node.Type(2), Op(5), Val(47)
  note: Entity Gate:
      | set to open when a positive signal value is passed into the control port. Closes when negative.
  note: Recieve signal from Chance-setting Server block for activation signal
  note: Service Time: 1700 Timestep
  note: Generates a single entity that causes Malicious Operation attack (entity generator) to generate one entity
  note: Sets MO_id up to 6 and resets to 1 for next Malicious Operation attack
  note: On Service Completion: Send a signal to data-logging SimFunctions
  note: Service Time: 610 Timestep
  Display : Display
  Entity Gate : EntityGate  InputPortMessageModes=m,m  OutputPortMessageModes=m
  Entity Generator : EntityGenerator  InputPortMessageModes=m  OutputPortMessageModes=m  GenerationMethod=Event-based  IntergenerationTimeAction=|  GenerateAction=|  AttributeName=MO_id  EntityType=Structured  EntityTypeName=MOAttack
      IntergenerationTimeAction=|
      | chanceDOS = rand(1,1);
      | if chanceDOS < 0.3
      |     dt = 1
      GenerateAction=|
      | persistent next_id_MO
      | 
      | if isempty(next_id_MO)
      |     next_id_MO = 1;
      |     %set seed for random number generation
      |     rng(12345);
      | end
      | 
      | entity.MO_id = next_id_MO
      | next_id_MO = next_id_MO + 1
      | 
      | if entity.MO_id == 1
      |     next_id_MO = 1
      settings: InputPortMap=u0
  Entity Server : EntityServer  InputPortMessageModes=m  OutputPortMessageModes=m  Capacity=1  ServiceTimeValue=1700  ServiceCompleteAction=|
      | sourceID(2); %vgr
      | sourceAddress(2); %/vgr_node
      | sourceType(5); %next task
      | sourceLocation(1); %Fischertechnik
      | destinationServiceAddress(1); %/hbw_node
      | destinationServiceType(1); %Motion Sensor
      | destinationServiceLocation(1); %FischerTechnik
      | accessedNodeAddress(3); 
      | accessedNodeType(2); %Boolean
      | operation(5); %write
      | value(47); %MO
  Entity Server1 : EntityServer  InputPortMessageModes=m  OutputPortMessageModes=m  Capacity=1  ServiceTimeValue=610  ServiceCompleteAction=|
      | sourceID(2); %vgr
      | sourceAddress(2); %/vgr_node
      | sourceType(5); %next task
      | sourceLocation(1); %Fischertechnik
      | destinationServiceAddress(1); %/hbw_node
      | destinationServiceType(1); %Motion Sensor
      | destinationServiceLocation(1); %FischerTechnik
      | accessedNodeAddress(3); 
      | accessedNodeType(2); %Boolean
      | operation(5); %write
      | value(47); %MO
  Entity Store : EntityStore  InputPortMessageModes=m  OutputPortMessageModes=m  Capacity=2
      settings: OutputPortMap=o4
  Entity Terminator1 : EntityTerminator  InputPortMessageModes=m  NumberEntitiesArrived=on
      settings: OutputPortMap=o0
  InitMaliciousOperation : Subsystem
  Malicious Operation : Subsystem  TreatAsAtomicUnit=on
  "Number of Entities Generated from main " : Display
  Simulink Function1 : Subsystem  TreatAsAtomicUnit=on
  Subsystem1 : Subsystem
  wires:
  Simulink Function1/1(Out1) -> Entity Generator/1
  Entity Terminator1/1 -> Display/1
  Entity Generator/1 -> Entity Store/1
  Entity Store/1 -> Entity Gate/2
  Entity Server/1 -> Entity Server1/1
  Malicious Operation/1(Out1) -> Entity Gate/1
  Subsystem1/1(Out1) -> Simulink Function1/1(In1)
  InitMaliciousOperation/1(Out1) -> "Number of Entities Generated from main "/1
  Entity Server1/1 -> Entity Terminator1/1
  Entity Gate/1 -> Entity Server/1
